simulink model "model_04"  (R2021b)
settings: Solver=ode45  StartTime=0  StopTime=100  RelTol=1e-3
settings Model: Creator=jimd  LastModifiedBy=jimd

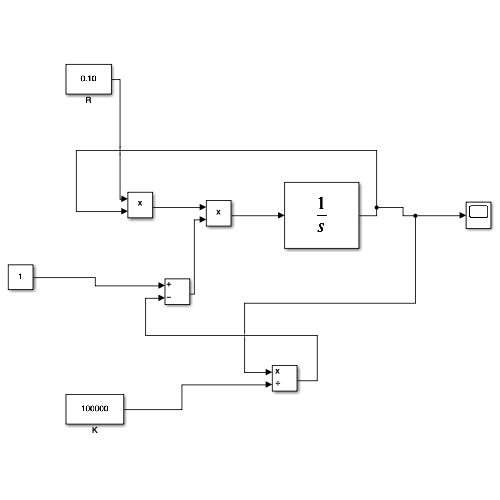
[thumbnail: Simulink's stored preview of the top-level diagram]
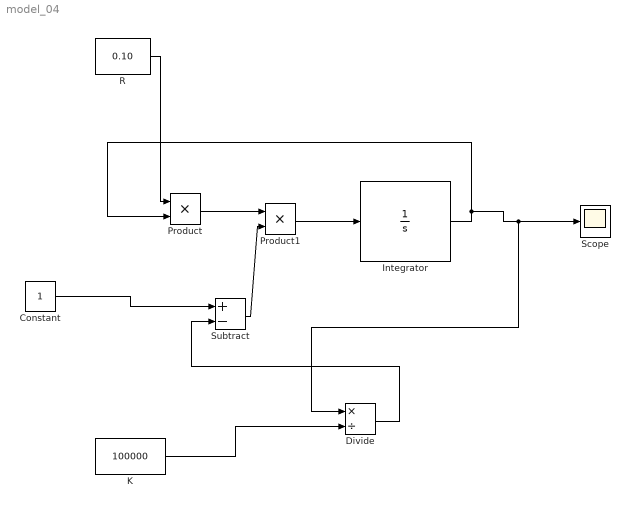
== system model_04 ==
  Constant : Constant
  Divide : Product  Inputs=*/
  Integrator : Integrator  InitialCondition=1000
  K : Constant  Value=100000
  Product : Product
  Product1 : Product
  R : Constant  Value=0.10
  Scope : Scope
  Subtract : Sum  Inputs=+-
  wires:
  R/1 -> Product/1
  Integrator/1 -> Product/2, Divide/1, Scope/1
  K/1 -> Divide/2
  Constant/1 -> Subtract/1
  Product/1 -> Product1/1
  Subtract/1 -> Product1/2
  Product1/1 -> Integrator/1
  Divide/1 -> Subtract/2
